simulink model "RobotX_IKin"  (R2024a)
settings: Solver=VariableStepAuto  StartTime=0.0  StopTime=10.0  MaxStep=1e-3  RelTol=1e-3
libraries: simulink x7, aerolibconvert2 x6, RobotX_Lib x2
settings Model: Creator=margaridaestrela  LastModifiedBy=margaridaestrela

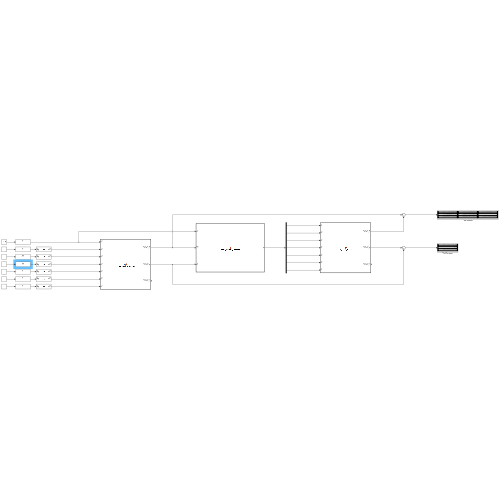
[thumbnail: Simulink's stored preview of the top-level diagram]
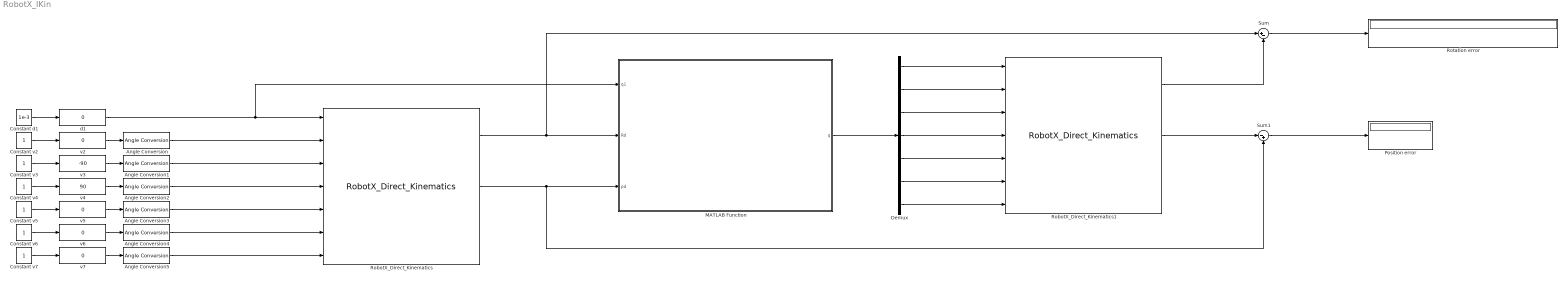
== system RobotX_IKin ==
  Angle Conversion{,1..5} (6 alike) : aerolibconvert2/Angle Conversion  IU=deg  OU=rad
  Constant d1 : Constant  Value=1e-3
  Constant v{2..7} (6 alike) : Constant
  Demux : Demux  Outputs=7
  MATLAB Function : MATLAB Function  TreatAsAtomicUnit=on
  Position error : Display
      settings: Format=decimal (Stored Integer)
  RobotX_Direct_Kinematics : RobotX_Lib/RobotX_Direct_Kinematics  SystemSampleTime=-1  VariantActivationTime=update diagram  AllowFlexibleInterface=on  Latency=0  AutoFrameSizeCalculation=off
  RobotX_Direct_Kinematics1 : RobotX_Lib/RobotX_Direct_Kinematics  SystemSampleTime=-1  VariantActivationTime=update diagram  AllowFlexibleInterface=on  Latency=0  AutoFrameSizeCalculation=off
  Rotation error : Display
      settings: Format=decimal (Stored Integer)
  Sum : Sum  Inputs=|+-
  Sum1 : Sum  Inputs=|-+
  d1 : simulink/Math Operations/Slider Gain  gain=0  low=-350  high=350
  v2 : simulink/Math Operations/Slider Gain  gain=0  low=-170  high=170
  v3 : simulink/Math Operations/Slider Gain  gain=-90  low=-190  high=45
  v4 : simulink/Math Operations/Slider Gain  gain=90  low=-120  high=156
  v5 : simulink/Math Operations/Slider Gain  gain=0  low=-185  high=185
  v6 : simulink/Math Operations/Slider Gain  gain=0  low=-120  high=120
  v7 : simulink/Math Operations/Slider Gain  gain=0  low=-350  high=350
  wires:
  Angle Conversion2/1 -> RobotX_Direct_Kinematics/4
  Constant v5/1 -> v5/1
  Angle Conversion/1 -> RobotX_Direct_Kinematics/2
  Angle Conversion1/1 -> RobotX_Direct_Kinematics/3
  v2/1 -> Angle Conversion/1
  RobotX_Direct_Kinematics/1 -> Sum/1, MATLAB Function/2(Rd)
  Angle Conversion3/1 -> RobotX_Direct_Kinematics/5
  d1/1 -> MATLAB Function/1(q1), RobotX_Direct_Kinematics/1
  Angle Conversion4/1 -> RobotX_Direct_Kinematics/6
  Constant v2/1 -> v2/1
  Constant v6/1 -> v6/1
  Constant d1/1 -> d1/1
  v5/1 -> Angle Conversion3/1
  v6/1 -> Angle Conversion4/1
  Constant v3/1 -> v3/1
  v3/1 -> Angle Conversion1/1
  RobotX_Direct_Kinematics/2 -> Sum1/2, MATLAB Function/3(pd)
  v4/1 -> Angle Conversion2/1
  Constant v4/1 -> v4/1
  Angle Conversion5/1 -> RobotX_Direct_Kinematics/7
  MATLAB Function/1(q) -> Demux/1
  Constant v7/1 -> v7/1
  v7/1 -> Angle Conversion5/1
  Demux/1 -> RobotX_Direct_Kinematics1/1
  Demux/2 -> RobotX_Direct_Kinematics1/2
  Demux/3 -> RobotX_Direct_Kinematics1/3
  Demux/4 -> RobotX_Direct_Kinematics1/4
  Demux/5 -> RobotX_Direct_Kinematics1/5
  Demux/6 -> RobotX_Direct_Kinematics1/6
  Demux/7 -> RobotX_Direct_Kinematics1/7
  RobotX_Direct_Kinematics1/1 -> Sum/2
  Sum/1 -> Rotation error/1
  RobotX_Direct_Kinematics1/2 -> Sum1/1
  Sum1/1 -> Position error/1

== matlab function RobotX_IKin/MATLAB Function ==
  data: q1 input; Rd input; q output; pd input
function q = RobotX_Inverse_Kinematics(q1, Rd, pd)
%Inverse Kinematics Estimation

q = zeros(1,7);

% Lengths
a2 = 25e-3;
a3 = 315e-3;
a4 = 35e-3;
d5 = 365e-3;
d7 = 80e-3;

z7 = Rd(:,3);
pw = pd - d7 * z7;

p1 = [-q1; 0; 189/250];
pw_ = pw - p1;

%% Solve v2
q2 = atan2(pw_(2,1), pw_(1,1));

%% Solve v4
%hypotenuse a4 -> d5
h45 = sqrt(a4^2 + d5^2);
q4 = asin(a4/h45);

%% Solve v3
p2 = [sin(q2)/40 - q1; cos(q2)/40; 189/250];
pw_ = pw - p2;

% p3 = [0;
%       (63*cos(q3))/200;
%       189/250 - (63*sin(q3))/200];

% p3 = pw - p1 - p2 - p4
p3 = pw_ - [-h45*sin(q4); -h45*cos(q4); -h45*cos(q4)];
c3 = p3(2,1)*200/63;
s3 = (189/250 - p3(3,1))*200/63;
q3 = atan2(s3,c3);


R0_4 = [sin(q3 + q4)*sin(q2), -cos(q2), -cos(q3 + q4)*sin(q2);
        sin(q3 + q4)*cos(q2),  sin(q2), -cos(q3 + q4)*cos(q2);
                cos(q3 + q4),        0,          sin(q3 + q4)];


%% Find R4_7
% R0_7 = R0_4 * R4_7
R4_7 = R0_4'* Rd;

% DKin(Robot(5:7,:))(1:3, 1:3)
% [                         -cos(q7)*sin(q6),                            -sin(q6)*sin(q7),          cos(q6)]
% [sin(q5)*sin(q7) - cos(q5)*cos(q6)*cos(q7), - cos(q7)*sin(q5) - cos(q5)*cos(q6)*sin(q7), -cos(q5)*sin(q6)]
% [cos(q5)*sin(q7) + cos(q6)*cos(q7)*sin(q5),   cos(q6)*sin(q5)*sin(q7) - cos(q5)*cos(q7),  sin(q5)*sin(q6)]

q5 = atan2(R4_7(3,3), -R4_7(2,3));
q6 = atan2(R4_7(2,3)/(-cos(q5)), R4_7(1,3));
q7 = atan2(R4_7(1,2), R4_7(1,1));

q = [q1, q2, q3, q4, q5, q6, q7];

end
